simulink subsystem "DCMotorModel"  (R2022a)
settings: Solver=VariableStepAuto  StartTime=0.0  StopTime=10.0  RelTol=1e-3
values from neighbouring files (symbols this model uses):
  Cshaft = 10    [SYDE351Project.m]
  If = 1.15    [SYDE351Project.m]
  Kb = 8*10^-3    (= 0.008)    [SYDE351Project.m]
  Kt = 8*10^-3    (= 0.008)    [SYDE351Project.m]
  La = 0.15*10^-3    (= 0.00015)    [SYDE351Project.m]
  Ra = 0.035    [SYDE351Project.m]
libraries: simulink x1
settings Model: Creator=Bronz  LastModifiedBy=Bronz

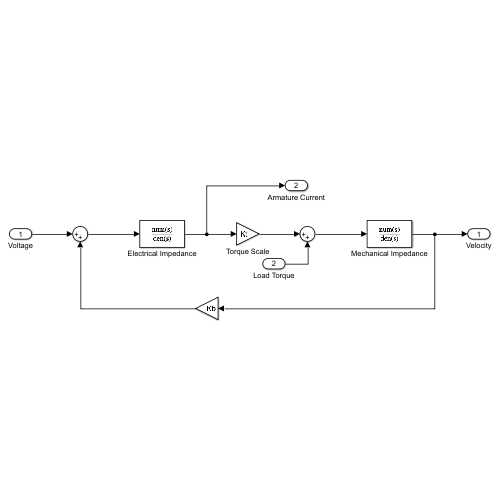
[thumbnail: Simulink's stored preview of the top-level diagram]
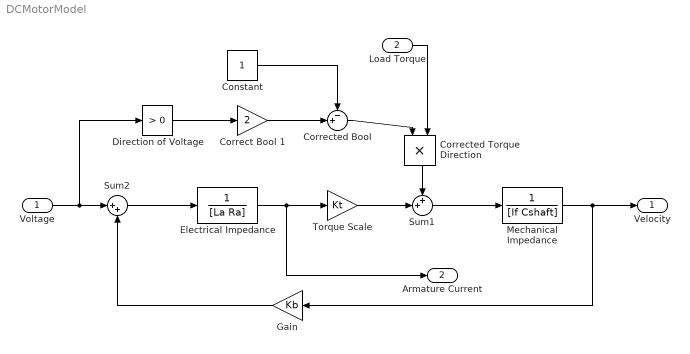
== system DCMotorModel ==
  Voltage : Inport
  Load Torque : Inport  Port=2
  Constant : Constant
  Correct Bool 1 : Gain  Gain=2
  Corrected Bool : Sum  Inputs=-+|
  Corrected Torque Direction : Product
  Direction of Voltage : simulink/Logic and Bit Operations/Compare To Zero  relop=>  OutDataTypeStr=boolean
  Electrical Impedance : TransferFcn  Denominator=[La Ra]
  Gain : Gain  Gain=Kb  ParamDataTypeStr=Inherit: Inherit from 'Gain'
  Mechanical Impedance : TransferFcn  Denominator=[If Cshaft]
  Sum1 : Sum  Inputs=++|
  Sum2 : Sum  Inputs=|++
  Torque Scale : Gain  Gain=Kt
  Velocity : Outport
  Armature Current : Outport  Port=2
  wires:
  Electrical Impedance/1 -> Armature Current/1, Torque Scale/1
  Voltage/1 -> Sum2/1, Direction of Voltage/1
  Sum2/1 -> Electrical Impedance/1
  Sum1/1 -> Mechanical Impedance/1
  Mechanical Impedance/1 -> Gain/1, Velocity/1
  Gain/1 -> Sum2/2
  Direction of Voltage/1 -> Correct Bool 1/1
  Load Torque/1 -> Corrected Torque Direction/2
  Torque Scale/1 -> Sum1/2
  Constant/1 -> Corrected Bool/1
  Correct Bool 1/1 -> Corrected Bool/2
  Corrected Torque Direction/1 -> Sum1/1
  Corrected Bool/1 -> Corrected Torque Direction/1
